simulink model "challenge-ENERGY SYSTEM-TSYP12"  (R2023b)
settings: Solver=VariableStepDiscrete  StartTime=0.0  StopTime=1  RelTol=1e-3
undefined symbols (not defined in the file): Ion, Lithium
libraries: spsCurrentMeasurementLib x2, spsSeriesRLCBranchLib x2, spsBatteryLib x1, spsControlledCurrentSourceLib x1, spsFuelCellStackLib x1, simulink x1, spsDiodeLib x1, spsMosfetLib x1, spspowerguiLib x1
settings Model: Creator=ADMIN  LastModifiedBy=rafed
settings SolverCC: AlgebraicLoopSolver=TrustRegion
settings DataIOCC: ReturnWorkspaceOutputs=off
settings DebuggingCC: UnconnectedInputMsg=warning  UnconnectedOutputMsg=warning  UnconnectedLineMsg=warning  ArithmeticOperatorsInVariantConditions=warning
settings ModelReferenceCC: EnableRefExpFcnMdlSchedulingChecks=on
settings SFSimCC: SimUseLocalCustomCode=off  CustomCodeUndefinedFunction=UseInterfaceOnly
settings RTWCC: RTWUseLocalCustomCode=off  DLArmComputeVersion=19.05

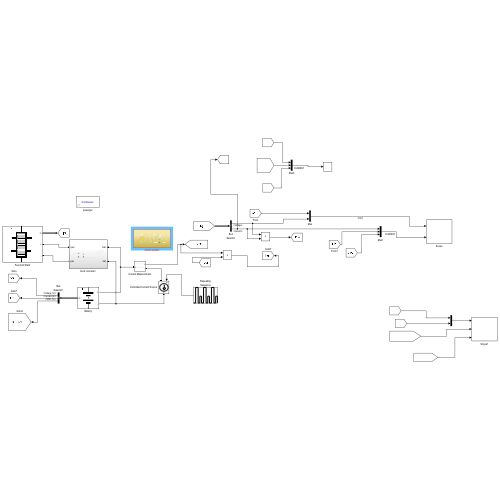
[thumbnail: Simulink's stored preview of the top-level diagram]
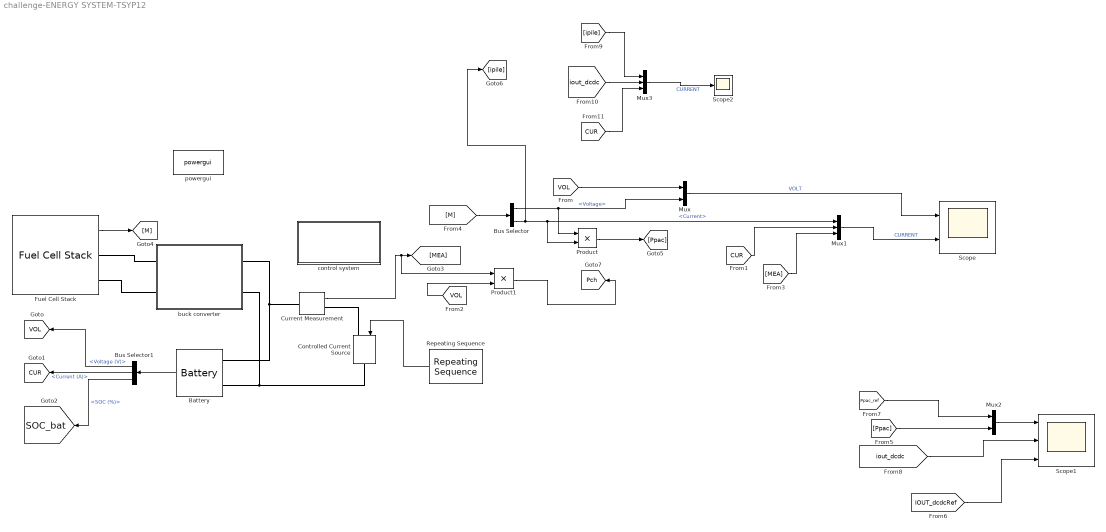
== system challenge-ENERGY SYSTEM-TSYP12 ==
  Battery : spsBatteryLib/Battery  BatType=Lithium-Ion  ShowTempParam=off  ThermalPreset=no  ShowAgeParam=off  NomV=24  NomQ=100  SOC=80  Batt_Tr=1  PresetModel=on  MaxQ=100  MinV=18  FullV=27.9357  Dis_rate=43.4783  R=0.0024  Normal_OP=90.4348  expZone="[25.9293      4.91304]"  current=[6.5 13 32.5]  Units=Time  Tci=20  NomT=20  T2=-30  MaxQ2=4.8  FullV2=7.1  Normal_OP2=5.655  expZone2="[6.58           1]"  Rca=0.6  ti=2000  Dp=0  Neq0=0  Tsim=1e6  Ta1=25  Qeol=5.4*0.9  Reol=0.013333*1.2  Char_age=[2.3478, 3]  Dis_age=[2.3478, 10]  N1=1500  N2=10500  N3=1000  N4=1400  Ta2=45  N5=950
      settings: LibrarySourceBlock=electricdrivelib/Extra Sources/Battery
  Bus Selector : BusSelector  OutputSignals=Voltage,Current
  Bus Selector1 : BusSelector  OutputSignals=Voltage (V),Current (A),SOC (%)
  Controlled Current Source : spsControlledCurrentSourceLib/Controlled Current Source  Initialize=on  Source_Type=AC  Amplitude=0  Phase=0  Frequency=0  Measurements=None
  Current Measurement : spsCurrentMeasurementLib/Current Measurement  PhasorSimulation=off  OutputType=Complex  PSBequivalent=0
  Fuel Cell Stack : spsFuelCellStackLib/Fuel Cell Stack  PresetModel=PEMFC - 1.26 kW - 24 Vdc  FcType=0  Detailed=Detailed  Eoc=[42,35]  NomVI=[52,24.23]  EndVI=[100,20]  Nc=42  n=46  TOp=55  AirFr=2400  SuppPress=[1.5,1]  Comp=[99.95,21,1]  SignX=off  SignY=off  FlowRateH2=off  FlowRateAir=off  SystemTemp=off  SystemPH2=off  SystemPAir=off  FCDyn=off  FC_tau=1  Peak_O2=80  V_Under=10
      settings: LibrarySourceBlock=electricdrivelib/Extra Sources/Fuel Cell Stack
  Mux : Mux  Inputs=2
  Mux1 : Mux  Inputs=3
  Mux2 : Mux  Inputs=2
  Mux3 : Mux  Inputs=3
  Product : Product
  Product1 : Product
  Repeating Sequence : simulink/Sources/Repeating Sequence  rep_seq_t=[0 2.999 3 6.999 7 9.4 9.4001 12]  rep_seq_y=[0 0 45 45 0 0 20 20]
  Scope : Scope  NumInputPorts=2
  Scope1 : Scope  NumInputPorts=3
  Scope2 : Scope
  "buck converter " : Subsystem
  control system : Subsystem
  powergui : spspowerguiLib/powergui  Priority=1  SimulationMode=Continuous  SampleTime=50e-6  frequency=60  Iterations=50  frequencyindice=0  Pbase=100e6  ErrMax=1e-4  UnitsV=kV  UnitsW=MW  buscounter=0  FunctionMessages=off  echomessages=off  EnableUseOfTLC=off  CurrentSourceSwitches=off  DisableSnubberDevices=off  DisableRonSwitches=off  DisableVfSwitches=off  DisplayEquations=off  AutomaticDiscreteSolvers=off  SolverType=Tustin/Backward Euler (TBE)  Interpol=off  ExternalGateDelay=off  methode=off  Ts=100  x0status=blocks  SPID=on  SwTol=0  HookPort=off  NonlinearTolerance=1e-4  nMaxIteration=100  ContinueOnMaxIteration=off  RestoreLinks=warning  ResistiveCurrentMeasurement=off  Frange=[0:2:500]  Ylog=off  Xlog=on  ShowGrid=off  save=off  variable=ZData  structure=0  ZoomFFT=off  StartTime=0.0  cycles=1  DisplayStyle=1  fundamental=60  FreqAxis=off  MaxFrequency=1000  frequencyindicesteady=1  RmsSteady=1  display=off
  tag scope: CUR=global, Pch=global, SOC_bat=global, VOL=global
  wires:
  Battery/1 -> Bus Selector1/1
  Bus Selector1/1 -> [VOL]  "<Voltage (V)>"
  [VOL] -> Mux/1
  Bus Selector/1 -> Product/1, Mux/2  "<Voltage>"
  Mux/1 -> Scope/1  "VOLT"
  Bus Selector/2 -> [ipile], Product/2, Mux1/1  "<Current>"
  Bus Selector1/2 -> [CUR]  "<Current (A)>"
  [CUR] -> Mux1/2
  Mux1/1 -> Scope/2  "CURRENT"
  Bus Selector1/3 -> [SOC_bat]  "<SOC (%)>"
  Current Measurement/1 -> Product1/1, [MEA]
  [MEA] -> Mux1/3
  Repeating Sequence/1 -> Controlled Current Source/1
  [M] -> Bus Selector/1
  Fuel Cell Stack/1 -> [M]
  Mux2/1 -> Scope1/1
  Product/1 -> [Ppac]
  [Ppac] -> Mux2/2
  [IOUT_dcdcRef] -> Scope1/3
  [Ppac_ref] -> Mux2/1
  [iout_dcdc] -> Scope1/2
  [iout_dcdc] -> Mux3/2
  [ipile] -> Mux3/1
  Mux3/1 -> Scope2/1  "CURRENT"
  [CUR] -> Mux3/3
  [VOL] -> Product1/2
  Product1/1 -> [Pch]
  connections:
  Current Measurement/LConn1 -- Battery/LConn1 -- "buck converter "/RConn1
  Controlled Current Source/RConn1 -- "buck converter "/RConn2 -- Battery/LConn2
  Current Measurement/RConn1 -- Controlled Current Source/LConn1
  Fuel Cell Stack/RConn1 -- "buck converter "/LConn1
  Fuel Cell Stack/RConn2 -- "buck converter "/LConn2

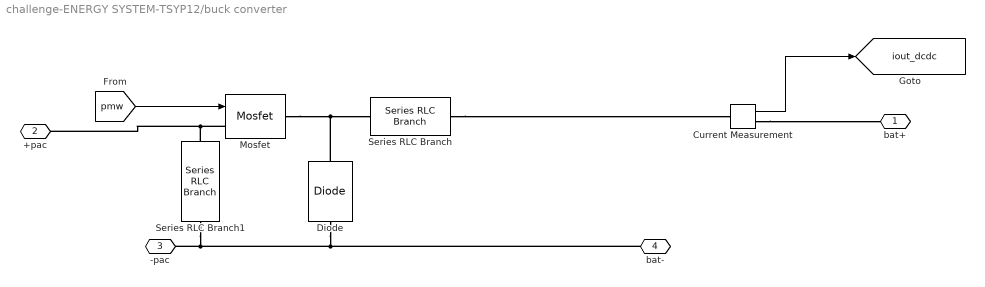
== system challenge-ENERGY SYSTEM-TSYP12/buck converter  ==
  Current Measurement : spsCurrentMeasurementLib/Current Measurement  PhasorSimulation=off  OutputType=Complex  PSBequivalent=0
  Diode : spsDiodeLib/Diode  Ron=0.001  Lon=0  Vf=0.8  IC=0  UseSnubber=0  Rs=500  Cs=250e-9  Measurements=off
  Mosfet : spsMosfetLib/Mosfet  Ron=0.1  Lon=0  Rd=0.01  Vfd=0  IC=0  Rs=1e5  Cs=inf  Measurements=off
  Series RLC Branch : spsSeriesRLCBranchLib/Series RLC Branch  LConnTagsString=__new0  RConnTagsString=__new0  BranchType=L  Resistance=1  Inductance=1e-3  SetiL0=off  InitialCurrent=0  Capacitance=1e-6  Setx0=off  InitialVoltage=0  Measurements=None
  Series RLC Branch1 : spsSeriesRLCBranchLib/Series RLC Branch  LConnTagsString=__new0  RConnTagsString=__new0  BranchType=C  Resistance=1  Inductance=1e-3  SetiL0=off  InitialCurrent=0  Capacitance=1000e-6  Setx0=on  InitialVoltage=42  Measurements=None
  bat+ : PMIOPort  Side=Right
  +pac : PMIOPort  Port=2  Side=Left
  -pac : PMIOPort  Port=3  Side=Left
  bat- : PMIOPort  Port=4  Side=Right
  tag scope: iout_dcdc=global
  wires:
  [pmw] -> Mosfet/1
  Current Measurement/1 -> [iout_dcdc]
  connections:
  Diode/LConn1 -- bat-/RConn1 -- Series RLC Branch1/RConn1 -- -pac/RConn1
  Mosfet/RConn1 -- Series RLC Branch/LConn1 -- Diode/RConn1
  Mosfet/LConn1 -- Series RLC Branch1/LConn1 -- +pac/RConn1
  Current Measurement/RConn1 -- bat+/RConn1
  Series RLC Branch/RConn1 -- Current Measurement/LConn1

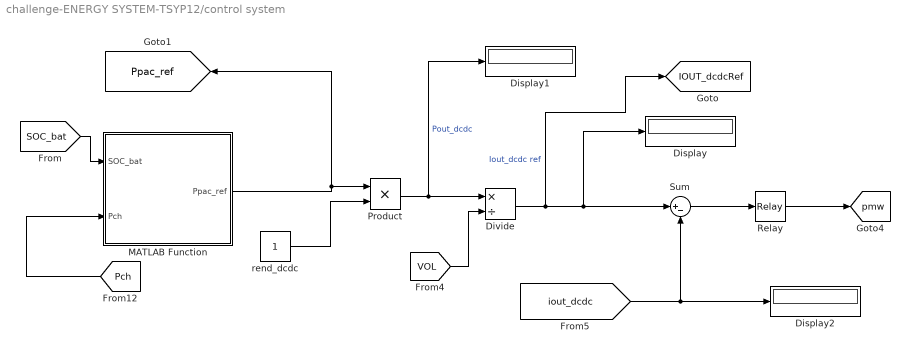
== system challenge-ENERGY SYSTEM-TSYP12/control system ==
  Display : Display
  Display1 : Display
  Display2 : Display
  Divide : Product  Inputs=*/
  MATLAB Function : MATLAB Function  TreatAsAtomicUnit=on
  Product : Product
  Relay : Relay  OnSwitchValue=0.5  OffSwitchValue=-0.5
  Sum : Sum  Inputs=|+-
  rend_dcdc : Constant
  tag scope: IOUT_dcdcRef=global, Ppac_ref=global, pmw=global
  wires:
  Product/1 -> Divide/1, Display1/1  "Pout_dcdc"
  Divide/1 -> [IOUT_dcdcRef], Display/1, Sum/1  "Iout_dcdc ref"
  Sum/1 -> Relay/1
  [VOL] -> Divide/2
  MATLAB Function/1(Ppac_ref) -> [Ppac_ref], Product/1
  rend_dcdc/1 -> Product/2
  Relay/1 -> [pmw]
  [iout_dcdc] -> Display2/1, Sum/2
  [SOC_bat] -> MATLAB Function/1(SOC_bat)
  [Pch] -> MATLAB Function/2(Pch)

== matlab function challenge-ENERGY SYSTEM-TSYP12/control system/MATLAB Function ==
  data: SOC_bat input; Ppac_ref output; Pch input
function Ppac_ref = func2(SOC_bat, Pch)
    % Determine Ppac_ref based on SOC_bat and Pch
    if Pch <= 0
        if SOC_bat <= 40
            Ppac_ref = 400;
        else
            Ppac_ref = 0;
        end
    else
        % Charging case
        if SOC_bat >= 80
            Ppac_ref = 0;
        elseif SOC_bat >= 60
            Ppac_ref = 100;
        elseif SOC_bat >= 40
            Ppac_ref = 200;
        else
            Ppac_ref = 400;
        end
    end
end
